simulink model "figure_1_7"  (R2026a)
settings: Solver=ode5  FixedStep=1e-4
settings Model: Creator=yagmu  LastModifiedBy=yagmu

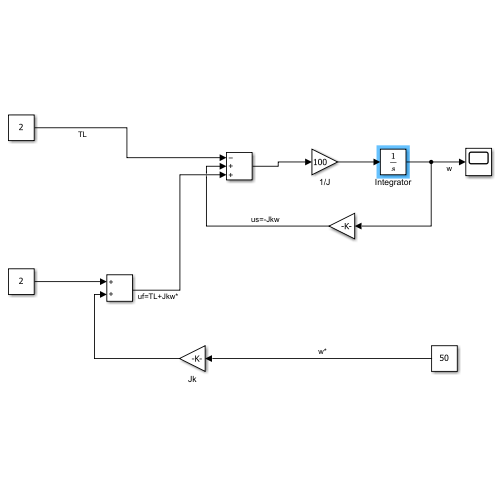
[thumbnail: Simulink's stored preview of the top-level diagram]
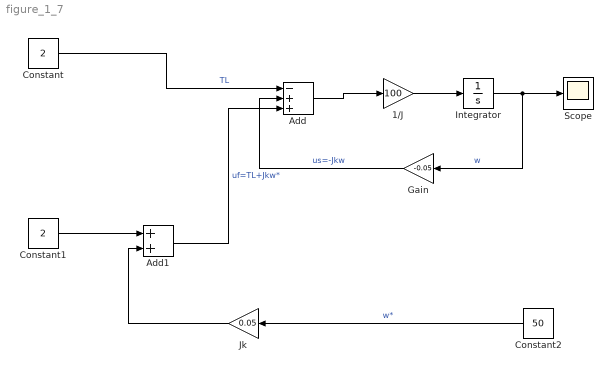
== system figure_1_7 ==
  1/J : Gain  Gain=100
  Add : Sum  Inputs=-++
  Add1 : Sum
  Constant : Constant  Value=2
  Constant1 : Constant  Value=2
  Constant2 : Constant  Value=50
  Gain : Gain  Gain=-0.05
  Integrator : Integrator
  Jk : Gain  Gain=0.05
  Scope : Scope
      settings: ActiveDisplayYMinimum=40  ActiveDisplayYMaximum=60
  wires:
  Constant/1 -> Add/1  "TL"
  Add/1 -> 1/J/1
  1/J/1 -> Integrator/1
  Integrator/1 -> Gain/1, Scope/1  "w"
  Constant1/1 -> Add1/1
  Add1/1 -> Add/3  "uf=TL+Jkw*"
  Jk/1 -> Add1/2
  Constant2/1 -> Jk/1  "w*"
  Gain/1 -> Add/2  "us=-Jkw"
